simulink model "electromecanico"  (R2022b)
settings: Solver=VariableStepAuto  StartTime=0.0  StopTime=10.0  RelTol=1e-3
values from neighbouring files (symbols this model uses):
  B = 12e-4    (= 0.0012)    [motorode.m]    (also in semode.m)
  J = 1e-3    (= 0.001)    [motorode.m]    (also in semode.m)
  Kt = 0.01    [motorode.m]    (also in semode.m)
  Kv = 0.01    [motorode.m]    (also in semode.m)
  L = 23e-3    (= 0.023)    [motorode.m]    (also in semode.m)
  R = 2    [motorode.m]    (also in semode.m)
settings Model: Creator=nemesis  LastModifiedBy=nemesis

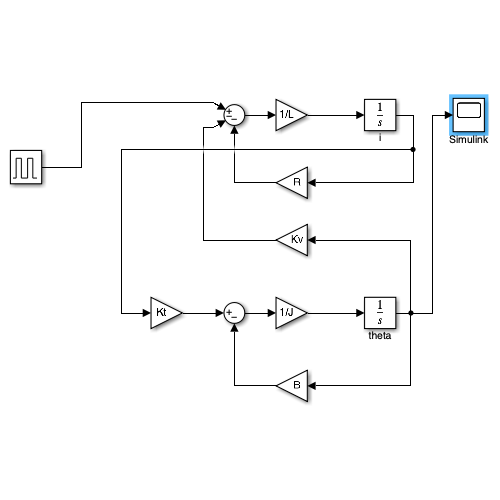
[thumbnail: Simulink's stored preview of the top-level diagram]
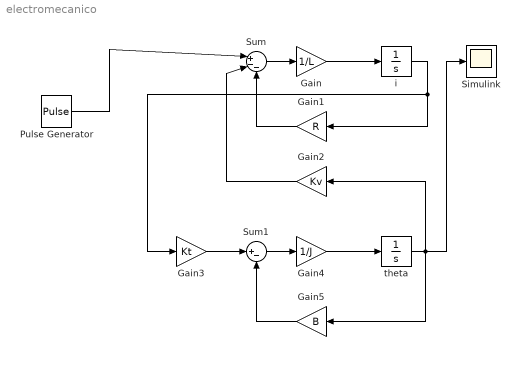
== system electromecanico ==
  Gain : Gain  Gain=1/L
  Gain1 : Gain  Gain=R
  Gain2 : Gain  Gain=Kv
  Gain3 : Gain  Gain=Kt
  Gain4 : Gain  Gain=1/J
  Gain5 : Gain  Gain=B
  Pulse Generator : DiscretePulseGenerator  PulseType=Time based  Amplitude=24  Period=1/20000  PulseWidth=25
  Simulink : Scope
  Sum : Sum  Inputs=|+--
  Sum1 : Sum  Inputs=|+-
  i : Integrator
  theta : Integrator
  wires:
  Sum/1 -> Gain/1
  Gain/1 -> i/1
  i/1 -> Gain1/1, Gain3/1
  Gain1/1 -> Sum/3
  Gain3/1 -> Sum1/1
  Gain5/1 -> Sum1/2
  Sum1/1 -> Gain4/1
  Gain4/1 -> theta/1
  theta/1 -> Simulink/1, Gain5/1, Gain2/1
  Gain2/1 -> Sum/2
  Pulse Generator/1 -> Sum/1
